simulink model "model_ex2"  (R2025b)
settings: Solver=VariableStepAuto  StartTime=0.0  StopTime=10.0  RelTol=1e-3
values from neighbouring files (symbols this model uses):
  d = 36.0    [mass_spring_damper_2.sldd]    (also in params_ex2.m = 36)
  F = 100.0    [mass_spring_damper_2.sldd]    (also in params_ex2.m = 100)
  k = 240.0    [mass_spring_damper_2.sldd]    (also in params_ex2.m = 240)
  m = 60.0    [mass_spring_damper_2.sldd]    (also in params_ex2.m = 60)
settings Model: DataDictionary=mass_spring_damper_2.sldd  Creator=mammadoo  LastModifiedBy=mammadoo

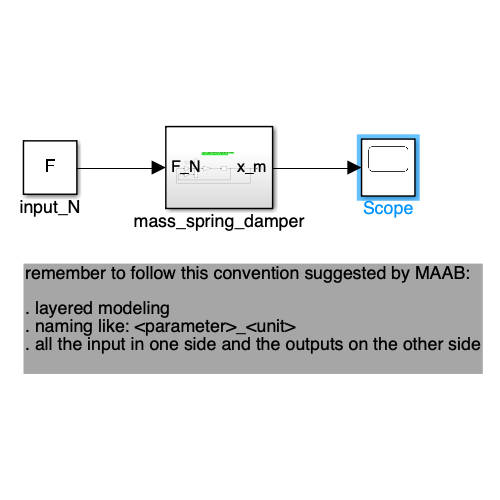
[thumbnail: Simulink's stored preview of the top-level diagram]
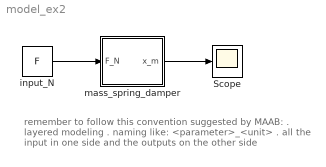
== system model_ex2 ==
  note: remember to follow this convention suggested by MAAB:
      |
      | . layered modeling
      | . naming like: <parameter>_<unit>
      | . all the input in one side and the outputs on the other side
  Scope : Scope
      settings: ActiveDisplayYMinimum=-0.083831870515023291  ActiveDisplayYMaximum=0.75448683463520971
  input_N : Constant  Value=F
  mass_spring_damper : Subsystem
  wires:
  input_N/1 -> mass_spring_damper/1(F_N)
  mass_spring_damper/1(x_m) -> Scope/1

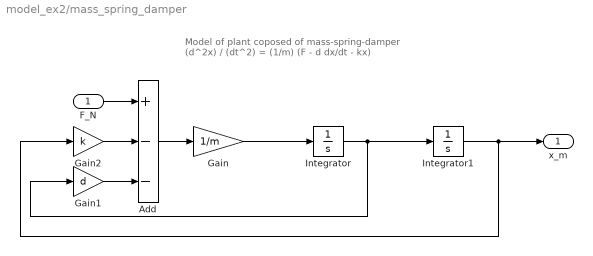
== system model_ex2/mass_spring_damper ==
  note: Model of plant coposed of mass-spring-damper
      | (d^2x) / (dt^2) = (1/m) (F - d dx/dt - kx)
  F_N : Inport
  Add : Sum  Inputs=+--
  Gain : Gain  Gain=1/m
  Gain1 : Gain  Gain=d
  Gain2 : Gain  Gain=k
  Integrator : Integrator
  Integrator1 : Integrator
  x_m : Outport
  wires:
  Add/1 -> Gain/1
  Gain/1 -> Integrator/1
  Gain2/1 -> Add/2
  F_N/1 -> Add/1
  Integrator/1 -> Gain1/1, Integrator1/1
  Gain1/1 -> Add/3
  Integrator1/1 -> x_m/1, Gain2/1
